simulink model "cxema2"  (R2014a)
settings: Solver=ode45  StartTime=0.0  StopTime=35  MaxStep=0.001  MinStep=0.0001  RelTol=1e-3
settings Model: Creator=User  LastModifiedBy=User

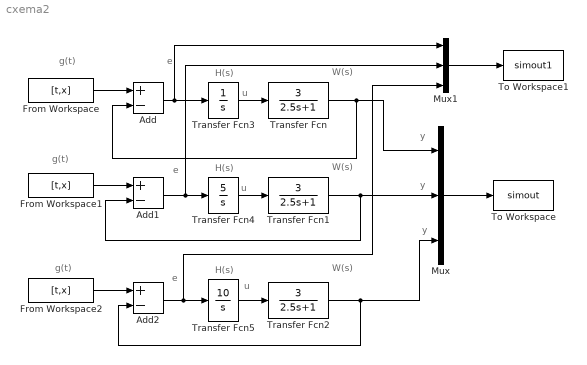
== system cxema2 ==
  note: W(s)
  note: W(s)
  note: W(s)
  note: H(s)
  note: H(s)
  note: H(s)
  note: u
  note: u
  note: u
  note: y
  note: y
  note: y
  note: g(t)
  note: g(t)
  note: g(t)
  note: e
  note: e
  note: e
  Add : Sum  Inputs=+-
  Add1 : Sum  Inputs=+-
  Add2 : Sum  Inputs=+-
  From Workspace : FromWorkspace  VariableName=[t,x]  SampleTime=0
  From Workspace1 : FromWorkspace  VariableName=[t,x]  SampleTime=0
  From Workspace2 : FromWorkspace  VariableName=[t,x]  SampleTime=0
  Mux : Mux  Inputs=3
  Mux1 : Mux  Inputs=3
  To Workspace : ToWorkspace  VariableName=simout  SaveFormat=Timeseries  SampleTime=-1
  To Workspace1 : ToWorkspace  VariableName=simout1  SaveFormat=Timeseries  SampleTime=-1
  Transfer Fcn : TransferFcn  Numerator=[3]  Denominator=[2.5 1]
  Transfer Fcn1 : TransferFcn  Numerator=[3]  Denominator=[2.5 1]
  Transfer Fcn2 : TransferFcn  Numerator=[3]  Denominator=[2.5 1]
  Transfer Fcn3 : TransferFcn  Denominator=[1 0]
  Transfer Fcn4 : TransferFcn  Numerator=[5]  Denominator=[1 0]
  Transfer Fcn5 : TransferFcn  Numerator=[10]  Denominator=[1 0]
  wires:
  Transfer Fcn3/1 -> Transfer Fcn/1
  Add/1 -> Mux1/1, Transfer Fcn3/1
  From Workspace/1 -> Add/1
  Transfer Fcn4/1 -> Transfer Fcn1/1
  Add1/1 -> Transfer Fcn4/1, Mux1/2
  From Workspace1/1 -> Add1/1
  Transfer Fcn5/1 -> Transfer Fcn2/1
  Add2/1 -> Mux1/3, Transfer Fcn5/1
  From Workspace2/1 -> Add2/1
  Transfer Fcn1/1 -> Mux/2, Add1/2
  Transfer Fcn/1 -> Add/2, Mux/1
  Transfer Fcn2/1 -> Add2/2, Mux/3
  Mux1/1 -> To Workspace1/1
  Mux/1 -> To Workspace/1
